simulink library "carnot"  (R2013b)
settings: Solver=ode45  StartTime=0.0  StopTime=10.0  RelTol=1e-3
undefined symbols (not defined in the file or in its folder): A, acol, Ahabit, Awin, Azimuth_Angle, AziWin, B, C, c1, c4, capc, caph, CarnotCallbacks_Density, CarnotCallbacks_Enthalpy, CarnotCallbacks_Enthalpy2Temperature, CarnotCallbacks_Entropy, CarnotCallbacks_Evaporation_Enthalpy, CarnotCallbacks_GlobalMessageLevel, CarnotCallbacks_Grashof, CarnotCallbacks_Heat_Capacity, CarnotCallbacks_Kinematic_Viscosity, CarnotCallbacks_Prandtl, CarnotCallbacks_Saturation_Property, CarnotCallbacks_Saturation_Temperature, CarnotCallbacks_Saturation_Value_Water, CarnotCallbacks_Specific_Volume, CarnotCallbacks_Thermal_Conductivity, CarnotCallbacks_Vapour_Content, CarnotCallbacks_Vapour_Pressure, con, cond, d, Dd, density, dfin, dia, DiameterLastPiece, DPConstant, dpipe, DPLinear, DPQuadratic, emission_out, fluid, FluidMix, FluidType, FPC, frame, g, GeodeticHeight, Gwin, heat_capacity, hgt, HP, Hroom, ID, inlet, K, l, lin, lpipe ... (+29)
undefined symbols (not defined in the file): c2, c3, c5, c6, cwall, dactive, height, mc, mID, rho, tau, UAneighbour, UAwall, uloss
libraries: carnot x333, simulink x25, simulink_extras x7
(part 13 of 16)

== system carnot/Storage/Thermal/Storage_Type_4_CONF ==
  Tamb : Inport
  THB_dhw : Inport  Port=2
  THB_bkpDHW : Inport  Port=3
  THB_hec : Inport  Port=4
  THB_sol : Inport  Port=5
  Storage_Type_4 : carnot/Storage/Thermal/Storage_Type_4  uloss=0.74  ubot=1.37  utop=0.74  cond=0.62  t0=tini  volume=0.75  dia=0.79  pos=standing cylinder  nconnect=4  nodes=50  mpoints=50
  T_Sensor_Surface : carnot/Control/T_Sensor_Surface  pos="[0.2         0.5         0.6]"  tdel=10  t0=tini(1)
  Sdat : Outport
  Tstg : Outport  Port=2
  THBdhw : Outport  Port=3
  THBbkpDHW : Outport  Port=4
  THBhec : Outport  Port=5
  THBsol : Outport  Port=6
  wires:
  Storage_Type_4/2 -> T_Sensor_Surface/1
  Storage_Type_4/1 -> Sdat/1
  THB_sol/1 -> Storage_Type_4/5  "THBsolar_in"
  THB_bkpDHW/1 -> Storage_Type_4/3  "THBbackup_in"
  THB_dhw/1 -> Storage_Type_4/2  "THBdhw_in"
  Tamb/1 -> Storage_Type_4/1
  Storage_Type_4/3 -> THBdhw/1
  Storage_Type_4/4 -> THBbkpDHW/1
  Storage_Type_4/6 -> THBsol/1
  Storage_Type_4/5 -> THBhec/1
  THB_hec/1 -> Storage_Type_4/4
  T_Sensor_Surface/1 -> Tstg/1

== system carnot/Storage/Thermal/Storage_Type_5 ==
  Tamb : Inport
  THB_dhw : Inport  Port=2
  THB_bkDHW : Inport  Port=3
  THB_heating : Inport  Port=4
  THB_bkHT : Inport  Port=5
  THB_solar : Inport  Port=6
  Bus Creator : BusCreator  Inputs=13
  Bus Creator1 : BusCreator  Inputs=2
  Demux : Demux  Outputs=2
  HX_EN12977_dhw : carnot/Storage/Thermal/Storage_Ports/HX_EN12977  h_in=0.02  h_out=0.95  ua0=642.2  uam=0.369  uat=0.684  dplin=100  dpqua=100  nodes=nodes  hgt=height  dia=dia
  HX_EN12977_solar : carnot/Storage/Thermal/Storage_Ports/HX_EN12977  h_in=0.45  h_out=0  ua0=678.6  uam=0.411  uat=0.287  dplin=100  dpqua=100  nodes=nodes  hgt=height  dia=dia
  pipe_bkp_dhw : carnot/Storage/Thermal/Storage_Ports/Pipe  h_in=1  h_out=0.45  nodes=nodes  hgt=height  dia=dia  dplin=10  dpqua=10
  pipe_bkp_heating : carnot/Storage/Thermal/Storage_Ports/Pipe  h_in=0.54  h_out=0.45  nodes=nodes  hgt=height  dia=dia  dplin=10  dpqua=10
  pipe_heating : carnot/Storage/Thermal/Storage_Ports/Pipe  h_in=0.45  h_out=0.54  nodes=nodes  hgt=height  dia=dia  dplin=10  dpqua=10
  select_T : Selector  InputPortWidth=nodes  IndexOptions=Index vector (dialog)  Indices=mpts  OutputSizes=1
  sfun_storageTnodes : carnot/Basic/Thermal_Models/sfun_storageTnodes  dia=dia  volume=volume  standing=standing  uloss=uloss  ubot=utop  utop=ubot  cond=cond  tini=tini  nodes=nodes  nconnect=nconnect
  Sdat : Outport
  T_nodes : Outport  Port=2
  THBdhw : Outport  Port=3
  THBbkDHW : Outport  Port=4
  THBheating : Outport  Port=5
  THBbkHT : Outport  Port=6
  THBsolar : Outport  Port=7
  wires:
  HX_EN12977_solar/2 -> Bus Creator/12, THBsolar/1  "THBsolar_out"
  THB_solar/1 -> Bus Creator/11, HX_EN12977_solar/2  "THBsolar_in"
  Bus Creator1/1 -> Bus Creator/2  "energy"
  Demux/2 -> Bus Creator1/2  "losses"
  Demux/1 -> Bus Creator1/1  "internal"
  pipe_bkp_dhw/1 -> sfun_storageTnodes/3
  pipe_bkp_dhw/2 -> THBbkDHW/1, Bus Creator/10  "THBother_out"
  THB_bkDHW/1 -> pipe_bkp_dhw/2, Bus Creator/9  "THBother_in"
  Bus Creator/1 -> Sdat/1
  sfun_storageTnodes/2 -> select_T/1, pipe_bkp_dhw/1, pipe_heating/1, HX_EN12977_solar/1, pipe_bkp_heating/1, HX_EN12977_dhw/1  "Tnodes"
  sfun_storageTnodes/1 -> Demux/1  "Energy"
  select_T/1 -> Bus Creator/13, T_nodes/1  "Tnodes"
  HX_EN12977_dhw/1 -> sfun_storageTnodes/2
  HX_EN12977_dhw/2 -> Bus Creator/4, THBdhw/1  "THBdhw_out"
  THB_dhw/1 -> Bus Creator/3, HX_EN12977_dhw/2  "THBdhw_in"
  Tamb/1 -> Bus Creator/1, sfun_storageTnodes/1  "Tamb"
  THB_heating/1 -> pipe_heating/2, Bus Creator/5  "THBheating_in"
  pipe_heating/1 -> sfun_storageTnodes/4
  pipe_heating/2 -> THBheating/1, Bus Creator/6  "THBheating_out"
  HX_EN12977_solar/1 -> sfun_storageTnodes/6
  THB_bkHT/1 -> pipe_bkp_heating/2, Bus Creator/7  "THBbackup_in"
  pipe_bkp_heating/1 -> sfun_storageTnodes/5
  pipe_bkp_heating/2 -> THBbkHT/1, Bus Creator/8  "THBbackup_out"

== system carnot/Storage/Thermal/Storage_Type_5_CONF ==
  Tamb : Inport
  THB_dhw : Inport  Port=2
  THB_bkpDHW : Inport  Port=3
  THB_hec : Inport  Port=4
  THB_bkpHec : Inport  Port=5
  THB_sol : Inport  Port=6
  Storage_Type_5 : carnot/Storage/Thermal/Storage_Type_5  uloss=0.74  ubot=1.37  utop=0.74  cond=0.62  t0=tini  volume=0.75  dia=0.79  pos=standing cylinder  nconnect=5  nodes=50  mpoints=50
  T_Sensor_Surface : carnot/Control/T_Sensor_Surface  pos=[0.1 0.5 0.7]  tdel=10  t0=tini(1)
  Sdat : Outport
  Tstg : Outport  Port=2
  THBdhw : Outport  Port=3
  THBbkpDHW : Outport  Port=4
  THBhec : Outport  Port=5
  THBbkpHec : Outport  Port=6
  THBsol : Outport  Port=7
  wires:
  T_Sensor_Surface/1 -> Tstg/1
  THB_bkpHec/1 -> Storage_Type_5/5
  Storage_Type_5/7 -> THBsol/1
  Storage_Type_5/4 -> THBbkpDHW/1
  Storage_Type_5/3 -> THBdhw/1
  Tamb/1 -> Storage_Type_5/1
  THB_dhw/1 -> Storage_Type_5/2  "THBdhw_in"
  THB_bkpDHW/1 -> Storage_Type_5/3  "THBbackup_in"
  THB_sol/1 -> Storage_Type_5/6  "THBsolar_in"
  Storage_Type_5/1 -> Sdat/1
  Storage_Type_5/2 -> T_Sensor_Surface/1
  Storage_Type_5/5 -> THBhec/1
  Storage_Type_5/6 -> THBbkpHec/1
  THB_hec/1 -> Storage_Type_5/4

== system carnot/Storage/Thermal/detailed_storage_models ==
  heat_exchanger_storage : Subsystem  mask(storage with heat exchanger){v=[0.002 0.0005], loss=0.1, uh=[500 1], uc=[500 1], uw=[300 1], mat=aluminium, m=[3 0.1], t0=20, dph=[200 100 1], dpc=[20 10 0.5], n=1}
      mask prompts: v "volume [exchanger storage] [m³]"; loss "ua losses [W/K]"; uh "heat transfer in exchanger [constant linear_in_massflow] [W/K]"; uc "heat transfer to storage [constant linear_massflow] [W/K]"; uw "heat transfer to wall [constant linear_in_massflow] [W/K]"; mat "material"; m "[mass_in_kg fraction_exchanger]"; t0 "initial temperature [degree centigrade]"; dph "pressure drop exchanger [linear quadratic lin_T] [Pa]"; dpc "pressure drop storage [linear quadratic lin_T] [Pa]"; n "number of nodes"
      mask help: This block is a heat exchanger, taking the fluid volume of the cold and hot side and the thermal capacity of the walls into account.
      mask init:
      | v = max(0.00001, v);
      | n = max(n,1);
      mask Help: web(fullfile(path_carnot('help'),'heat_exchanger_storage.html'),'-helpbrowser')
      mask TypeOptions mat: aluminium | bronze | cast iron | steel | stainless steel | copper | brass | gravel | granite | glass | PU-foam | glass wool
      mask Display: plot(0,-10,110,95,[30,30,35,65,70,70,65,35,30],[90,60,54,54,60,90,95,95,90],[30,66,34,66,34,66,30],[63,63,68,73,76,81,81])

== system carnot/Storage/Thermal/surface_models ==
  Isolated_Cover : Subsystem  mask(isolated cover){u=0.6}
      mask prompts: u "loss coefficient of isolation [W/(m²*K)]"
      mask help: This is a surface-model for ground storages. It describes the absorption of solar radiation and the heat losses by wind.
      mask Help: web(fullfile(path_carnot('help'),'Isolated_Cover.html'),'-helpbrowser')
  Open_Surface : Subsystem  mask(open surface){albedo=0.6}
      mask prompts: albedo "albedo of the surface [0..1]"
      mask help: This is a surface-model for ground storages. It describes the absorption of solar radiation and the heat losses by wind.
      mask init:
      | albedo = min(1, max(0, albedo));
      mask Help: web(fullfile(path_carnot('help'),'Open_Surface.html'),'-helpbrowser')

== system carnot/Basic/Hydraulics/Flow_Mixer_basic/average_1 ==
  In1 : Inport
  In2 : Inport  Port=2
  average2 : Gain  Gain=0.5  SaturateOnIntegerOverflow=on  OutDataTypeStr=Inherit: Same as input  ParamDataTypeStr=Inherit: Same as input
  sum2 : Sum  SaturateOnIntegerOverflow=on  InputSameDT=on  OutDataTypeStr=Inherit: Same as first input
  Out1 : Outport
  wires:
  In1/1 -> sum2/1
  average2/1 -> Out1/1
  sum2/1 -> average2/1
  In2/1 -> sum2/2

== system carnot/Basic/Hydraulics/Flow_Mixer_basic/decrease_ID1 ==
  In1 : Inport
  Abs : Abs
  Bias : Bias  Bias=-1
  Dot Product1 : DotProduct  InputSameDT=on  OutDataTypeStr=Inherit: Inherit via internal rule
  Sign : Signum
  Out1 : Outport
  wires:
  Bias/1 -> Dot Product1/2
  Sign/1 -> Dot Product1/1
  Abs/1 -> Bias/1
  Dot Product1/1 -> Out1/1
  In1/1 -> Sign/1, Abs/1

== system carnot/Basic/Hydraulics/Flow_Mixer_basic/decrease_ID2 ==
  In1 : Inport
  Abs : Abs
  Bias : Bias  Bias=-1
  Dot Product1 : DotProduct  InputSameDT=on  OutDataTypeStr=Inherit: Inherit via internal rule
  Sign : Signum
  Out1 : Outport
  wires:
  In1/1 -> Abs/1, Sign/1
  Dot Product1/1 -> Out1/1
  Abs/1 -> Bias/1
  Sign/1 -> Dot Product1/1
  Bias/1 -> Dot Product1/2

== system carnot/Basic/Hydraulics/Mix_T_Mdot/select1 ==
  In1 : Inport
  Bus Selector1 : BusSelector  OutputSignals=Temperature,MassFlow,Pressure,FluidType,FluidMix
  Mux : Mux  Inputs=5
  Out1 : Outport
  wires:
  Mux/1 -> Out1/1
  In1/1 -> Bus Selector1/1
  Bus Selector1/5 -> Mux/5  "<FluidMix>"
  Bus Selector1/4 -> Mux/4  "<FluidType>"
  Bus Selector1/3 -> Mux/3  "<Pressure>"
  Bus Selector1/2 -> Mux/2  "<MassFlow>"
  Bus Selector1/1 -> Mux/1  "<Temperature>"

== system carnot/Basic/Hydraulics/Mix_T_Mdot/select2 ==
  In1 : Inport
  Bus Selector1 : BusSelector  OutputSignals=Temperature,MassFlow,Pressure,FluidType,FluidMix
  Mux : Mux  Inputs=5
  Out1 : Outport
  wires:
  Bus Selector1/1 -> Mux/1  "<Temperature>"
  Bus Selector1/2 -> Mux/2  "<MassFlow>"
  Bus Selector1/3 -> Mux/3  "<Pressure>"
  Bus Selector1/4 -> Mux/4  "<FluidType>"
  Bus Selector1/5 -> Mux/5  "<FluidMix>"
  In1/1 -> Bus Selector1/1
  Mux/1 -> Out1/1

== system carnot/Basic/Pressure_Drop/Pressure_Drop_Fix/c_calc ==
  Enable : EnablePort
  Constant : Constant  Value=con
  con : Outport  InitialOutput=con
  wires:
  Constant/1 -> con/1

== system carnot/Basic/Pressure_Drop/Pressure_Drop_Fix/lq_calc ==
  Enable : EnablePort
  Constant : Constant  Value=lin
  Constant1 : Constant  Value=qua
  Out1 : Outport  InitialOutput=lin
  Out2 : Outport  Port=2  InitialOutput=qua
  wires:
  Constant/1 -> Out1/1
  Constant1/1 -> Out2/1

== system carnot/Basic/Pressure_Drop/Pressure_Drop_PipeTheory/DP_Geometry ==
  Tnodes : Inport
  mdot : Inport  Port=2
  Enable : EnablePort
  Bus Selector4 : BusSelector  OutputSignals=MassFlow,Pressure,FluidType,FluidMix
  S-Function : S-Function  FunctionName=pipe_PressureDrop  Parameters="dia, len,  rough, nbend"  EnableBusSupport=off
  lin : Outport  OutputWhenDisabled=reset  InitialOutput=0
  qua : Outport  Port=2  OutputWhenDisabled=reset  InitialOutput=0
  dp : Outport  Port=3  OutputWhenDisabled=reset  InitialOutput=0
  wires:
  Tnodes/1 -> S-Function/1
  S-Function/1 -> lin/1
  S-Function/2 -> qua/1
  mdot/1 -> Bus Selector4/1
  Bus Selector4/1 -> S-Function/2  "<MassFlow>"
  Bus Selector4/2 -> S-Function/3  "<Pressure>"
  Bus Selector4/3 -> S-Function/4  "<FluidType>"
  Bus Selector4/4 -> S-Function/5  "<FluidMix>"
  S-Function/3 -> dp/1

== system carnot/Basic/Pressure_Drop/Pressure_Drop_changeD/2//pi//d^2//density ==
  note: dp = ceta * density/2 *v^2
      | for Dlast > Dhere : ceta = (1 - D_last/D_here)^2
      | v = mdot/A/density
      | dp = ceta * mdot^2 / 2 / A^2 / densitiy
      | with A = pi/4*d^2
      | dp = 8*mdot^2/pi^2/d^4/denstiy
      | dp=qua*mdot^2
      | qua = 8/(pi^2*density) * ceta / d^4
  THB : Inport
  Enable : EnablePort
  Bus Selector3 : BusSelector  OutputSignals=DiameterLastPiece
  Density : carnot/Basic/Material_Properties/Density  VariantControl=CarlibClassic  INPUTARGUMENTS=THB  DEBUGLEVEL=DEBUGLEVEL  MAXTOTALWARNINGS=inf  MAXCONSECUTIVEWARNINGS=inf  WRITETOFILE=0  FILENAME='errors.txt'
  Gain : Gain  Gain=pi^2/8
  Gain1 : Gain  Gain=1/dia
  Lookup Table : Lookup  InputValues=[0:0.05:1, 10, 100]  Table="[(1 - [0:0.05:1]).^2,  1.2, 1.2]"
  Math Function2 : Math  Operator=square  SaturateOnIntegerOverflow=on
  Math Function3 : Math  Operator=square  SaturateOnIntegerOverflow=on
  Product : Product  Inputs=/*/  RndMeth=Zero
  min(Dlast,dia) : Saturate  UpperLimit=dia  LowerLimit=0
  qua : Outport
  wires:
  Density/1 -> Gain/1
  THB/1 -> Bus Selector3/1, Density/1
  Bus Selector3/1 -> Gain1/1, min(Dlast,dia)/1  "<DiameterLastPiece>"
  Gain/1 -> Product/1
  Product/1 -> qua/1
  Gain1/1 -> Lookup Table/1  "Dlast/D"
  min(Dlast,dia)/1 -> Math Function2/1
  Math Function2/1 -> Math Function3/1
  Math Function3/1 -> Product/3
  Lookup Table/1 -> Product/2  "ceta"

== system carnot/Basic/Pressure_Drop/Pressure_Drop_staticHeight/Density_x_Gravity ==
  Tnodes : Inport
  THB : Inport  Port=2
  height : Inport  Port=3
  Enable : EnablePort
  Add : Sum
  Add1 : Sum  Inputs=1
  Bus Selector4 : BusSelector  OutputSignals=Pressure,FluidType,FluidMix,GeodeticHeight
  Constant : Constant  Value=9.81
  Density : carnot/Basic/Material_Properties/Density  VariantControl=CarlibClassic  INPUTARGUMENTS=state variables (classic)  DEBUGLEVEL=DEBUGLEVEL  MAXTOTALWARNINGS=inf  MAXCONSECUTIVEWARNINGS=inf  WRITETOFILE=0  FILENAME='errors.txt'
  Product : Product  Inputs=/***  RndMeth=Zero
  Width : Width
  pstat : Outport
  GeodeticHeight : Outport  Port=2
  wires:
  Add1/1 -> pstat/1
  Constant/1 -> Product/3
  Product/1 -> Add1/1
  Density/1 -> Product/4
  Width/1 -> Product/1
  Add/1 -> GeodeticHeight/1
  height/1 -> Product/2, Add/2
  Bus Selector4/4 -> Add/1  "<GeodeticHeight>"
  Tnodes/1 -> Width/1, Density/1
  THB/1 -> Bus Selector4/1
  Bus Selector4/3 -> Density/4  "<FluidMix>"
  Bus Selector4/2 -> Density/3  "<FluidType>"
  Bus Selector4/1 -> Density/2  "<Pressure>"

== system carnot/Basic/Thermal_Models/Combustion_Calculation/exhaust gas ==
  note: gas = 1
      | liquid = 2
      | solid = 3
  ID : Inport
  h : Inport  Port=2
  c : Inport  Port=3
  o : Inport  Port=4
  s : Inport  Port=5
  n : Inport  Port=6
  w : Inport  Port=7
  Demux : Demux
  Multiport Switch : MultiPortSwitch  SaturateOnIntegerOverflow=on  InputSameDT=on
  Terminator : Terminator
  fluid/solid : Subsystem
  gas : Subsystem
  CO2 : Outport
  H2O : Outport  Port=2
  SO2 : Outport  Port=3
  N2 : Outport  Port=4
  wires:
  ID/1 -> Multiport Switch/1
  fluid/solid/1(Out1) -> Multiport Switch/4, Multiport Switch/3
  Multiport Switch/1 -> Demux/1
  Demux/4 -> N2/1
  Demux/3 -> SO2/1
  Demux/2 -> H2O/1
  Demux/1 -> CO2/1
  s/1 -> gas/3(s), fluid/solid/3(s)
  n/1 -> gas/4(n), fluid/solid/4(n)
  h/1 -> gas/2(h), fluid/solid/2(h)
  c/1 -> gas/1(c), fluid/solid/1(c)
  o/1 -> Terminator/1
  w/1 -> fluid/solid/5(w)
  gas/1(Out1) -> Multiport Switch/2

== system carnot/Basic/Thermal_Models/HeatPump_basic/P_el calculus ==
  note: Pel = K4*Tcold_in + K5*Thot_out + K6
  Thot_out : Inport
  Tcold_in : Inport  Port=2
  Add : Sum  Inputs=+++
  Thot_dependancy : Gain  Gain=K(5)  SaturateOnIntegerOverflow=on  OutDataTypeStr=Inherit: Same as input  ParamDataTypeStr=Inherit: Same as input
  Tsource dependancy : Gain  Gain=K(4)  SaturateOnIntegerOverflow=on  OutDataTypeStr=Inherit: Same as input  ParamDataTypeStr=Inherit: Same as input
  constant power : Constant  Value=K(6)
  P_el : Outport
  wires:
  Thot_dependancy/1 -> Add/1
  Thot_out/1 -> Thot_dependancy/1
  Tsource dependancy/1 -> Add/2
  Add/1 -> P_el/1
  Tcold_in/1 -> Tsource dependancy/1
  constant power/1 -> Add/3

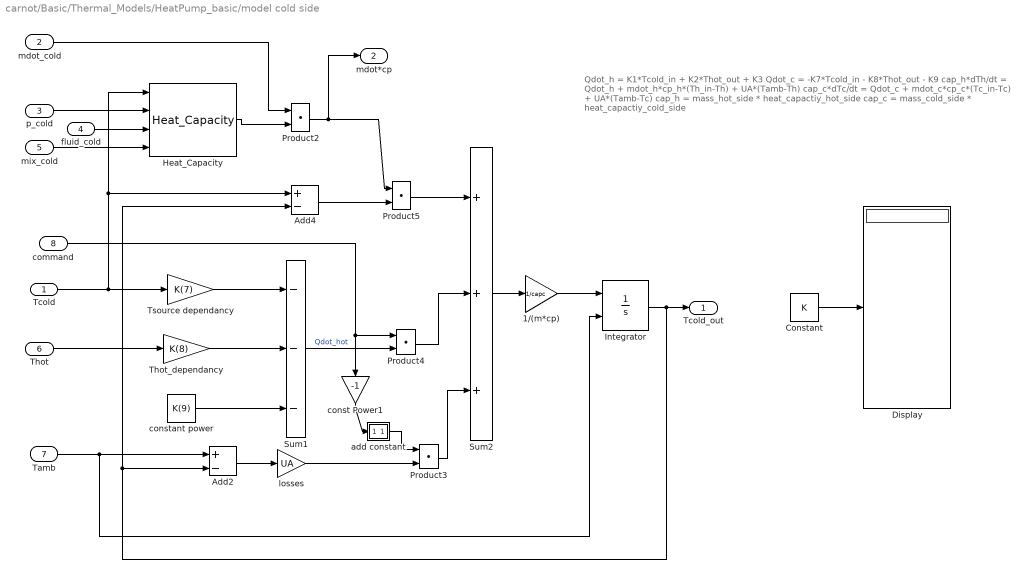
== system carnot/Basic/Thermal_Models/HeatPump_basic/model cold side ==
  note: Qdot_h = K1*Tcold_in + K2*Thot_out + K3
      |
      | Qdot_c = -K7*Tcold_in - K8*Thot_out - K9
      |
      | cap_h*dTh/dt = Qdot_h + mdot_h*cp_h*(Th_in-Th) + UA*(Tamb-Th)
      |
      | cap_c*dTc/dt = Qdot_c + mdot_c*cp_c*(Tc_in-Tc) + UA*(Tamb-Tc)
      |
      | cap_h = mass_hot_side * heat_capactiy_hot_side
      |
      | cap_c = mass_cold_side * heat_capactiy_cold_side
  Tcold : Inport
  mdot_cold : Inport  Port=2
  p_cold : Inport  Port=3
  fluid_cold : Inport  Port=4
  mix_cold : Inport  Port=5
  Thot : Inport  Port=6
  Tamb : Inport  Port=7
  command : Inport  Port=8
  1/(m*cp) : Gain  Gain=1/capc
  Add2 : Sum  Inputs=+-
  Add4 : Sum  Inputs=+-
  Constant : Constant  Value=K
  Display : Display
  Heat_Capacity : carnot/Basic/Material_Properties/Heat_Capacity  VariantControl=CarlibClassic  INPUTARGUMENTS=state variables (classic)  DEBUGLEVEL=DEBUGLEVEL  MAXTOTALWARNINGS=inf  MAXCONSECUTIVEWARNINGS=inf  WRITETOFILE=0  FILENAME='errors.txt'
  Integrator : Integrator  InitialConditionSource=external  InitialCondition=25
  Product{2..5} (4 alike) : DotProduct  InputSameDT=on  OutDataTypeStr=Inherit: Inherit via internal rule
  Sum1 : Sum  Inputs=---  SaturateOnIntegerOverflow=on  InputSameDT=on  OutDataTypeStr=Inherit: Same as first input
  Sum2 : Sum  Inputs=3  SaturateOnIntegerOverflow=on  InputSameDT=on  OutDataTypeStr=Inherit: Same as first input
  Thot_dependancy : Gain  Gain=K(8)  SaturateOnIntegerOverflow=on  OutDataTypeStr=Inherit: Same as input  ParamDataTypeStr=Inherit: Same as input
  Tsource dependancy : Gain  Gain=K(7)  SaturateOnIntegerOverflow=on  OutDataTypeStr=Inherit: Same as input  ParamDataTypeStr=Inherit: Same as input
  add constant : Subsystem  mask(add constant){c=+1}
      mask prompts: c "constant c"
      mask help: This block adds a constant c to each element of the input vector.
      mask Help: eval('htmlhelp (''chap_4_2a.htm#add_constant'')')
      mask Display: disp('+c');
  const Power1 : Gain  Gain=-1  SaturateOnIntegerOverflow=on  OutDataTypeStr=Inherit: Same as input  ParamDataTypeStr=Inherit: Same as input
  constant power : Constant  Value=K(9)
  losses : Gain  Gain=UA
  Tcold_out : Outport
  mdot*cp : Outport  Port=2
  wires:
  Constant/1 -> Display/1
  1/(m*cp)/1 -> Integrator/1
  fluid_cold/1 -> Heat_Capacity/3
  mix_cold/1 -> Heat_Capacity/4
  p_cold/1 -> Heat_Capacity/2
  Thot/1 -> Thot_dependancy/1
  Product2/1 -> mdot*cp/1, Product5/1
  Heat_Capacity/1 -> Product2/2
  mdot_cold/1 -> Product2/1
  Add2/1 -> losses/1
  Tcold/1 -> Add4/1, Heat_Capacity/1, Tsource dependancy/1
  Tsource dependancy/1 -> Sum1/1
  Thot_dependancy/1 -> Sum1/2
  constant power/1 -> Sum1/3
  Sum1/1 -> Product4/2  "Qdot_hot"
  Tamb/1 -> Add2/1, Integrator/2
  command/1 -> Product4/1, const Power1/1
  losses/1 -> Product3/2
  add constant/1(Out1) -> Product3/1
  const Power1/1 -> add constant/1(In1)
  Add4/1 -> Product5/2
  Sum2/1 -> 1/(m*cp)/1
  Product3/1 -> Sum2/3
  Product4/1 -> Sum2/2
  Product5/1 -> Sum2/1
  Integrator/1 -> Tcold_out/1, Add2/2, Add4/2

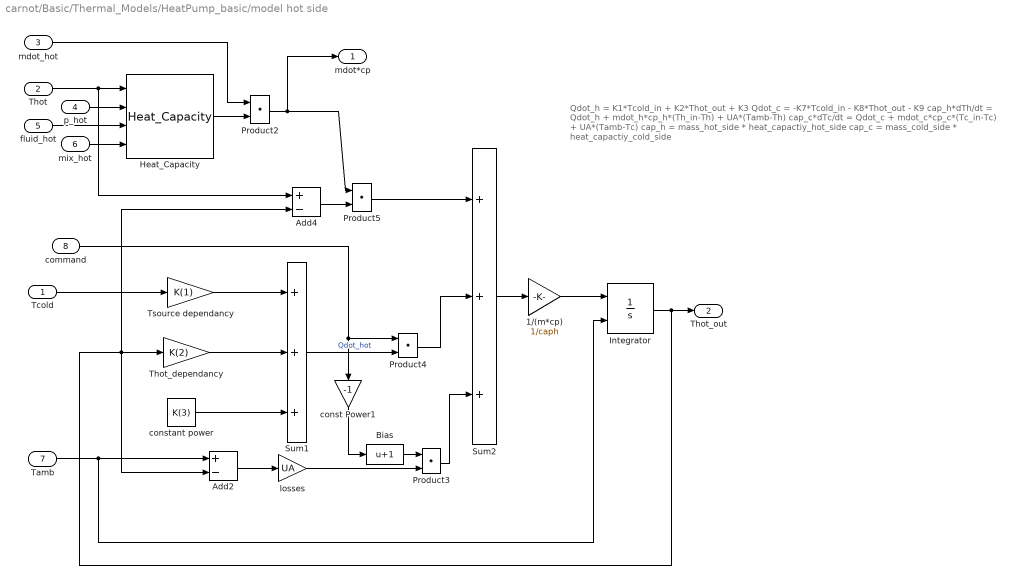
== system carnot/Basic/Thermal_Models/HeatPump_basic/model hot side ==
  note: Qdot_h = K1*Tcold_in + K2*Thot_out + K3
      |
      | Qdot_c = -K7*Tcold_in - K8*Thot_out - K9
      |
      | cap_h*dTh/dt = Qdot_h + mdot_h*cp_h*(Th_in-Th) + UA*(Tamb-Th)
      |
      | cap_c*dTc/dt = Qdot_c + mdot_c*cp_c*(Tc_in-Tc) + UA*(Tamb-Tc)
      |
      | cap_h = mass_hot_side * heat_capactiy_hot_side
      |
      | cap_c = mass_cold_side * heat_capactiy_cold_side
  Tcold : Inport
  Thot : Inport  Port=2
  mdot_hot : Inport  Port=3
  p_hot : Inport  Port=4
  fluid_hot : Inport  Port=5
  mix_hot : Inport  Port=6
  Tamb : Inport  Port=7
  command : Inport  Port=8
  1/(m*cp) : Gain  Gain=1/caph
  Add2 : Sum  Inputs=+-
  Add4 : Sum  Inputs=+-
  Bias : Bias  Bias=1
  Heat_Capacity : carnot/Basic/Material_Properties/Heat_Capacity  VariantControl=CarlibClassic  INPUTARGUMENTS=state variables (classic)  DEBUGLEVEL=DEBUGLEVEL  MAXTOTALWARNINGS=inf  MAXCONSECUTIVEWARNINGS=inf  WRITETOFILE=0  FILENAME='errors.txt'
  Integrator : Integrator  InitialConditionSource=external  InitialCondition=25
  Product{2..5} (4 alike) : DotProduct  InputSameDT=on  OutDataTypeStr=Inherit: Inherit via internal rule
  Sum1 : Sum  Inputs=+++  SaturateOnIntegerOverflow=on  InputSameDT=on  OutDataTypeStr=Inherit: Same as first input
  Sum2 : Sum  Inputs=+++  SaturateOnIntegerOverflow=on  InputSameDT=on  OutDataTypeStr=Inherit: Same as first input
  Thot_dependancy : Gain  Gain=K(2)  SaturateOnIntegerOverflow=on  OutDataTypeStr=Inherit: Same as input  ParamDataTypeStr=Inherit: Same as input
  Tsource dependancy : Gain  Gain=K(1)  SaturateOnIntegerOverflow=on  OutDataTypeStr=Inherit: Same as input  ParamDataTypeStr=Inherit: Same as input
  const Power1 : Gain  Gain=-1  SaturateOnIntegerOverflow=on  OutDataTypeStr=Inherit: Same as input  ParamDataTypeStr=Inherit: Same as input
  constant power : Constant  Value=K(3)
  losses : Gain  Gain=UA
  mdot*cp : Outport
  Thot_out : Outport  Port=2
  wires:
  Integrator/1 -> Add2/2, Thot_dependancy/1, Add4/2, Thot_out/1
  Product5/1 -> Sum2/1
  Product4/1 -> Sum2/2
  Product3/1 -> Sum2/3
  1/(m*cp)/1 -> Integrator/1
  Sum2/1 -> 1/(m*cp)/1
  Add4/1 -> Product5/2
  const Power1/1 -> Bias/1
  Bias/1 -> Product3/1
  losses/1 -> Product3/2
  command/1 -> const Power1/1, Product4/1
  Tamb/1 -> Integrator/2, Add2/1
  Sum1/1 -> Product4/2  "Qdot_hot"
  constant power/1 -> Sum1/3
  Thot_dependancy/1 -> Sum1/2
  Tsource dependancy/1 -> Sum1/1
  Tcold/1 -> Tsource dependancy/1
  Add2/1 -> losses/1
  mdot_hot/1 -> Product2/1
  Heat_Capacity/1 -> Product2/2
  Product2/1 -> Product5/1, mdot*cp/1
  Thot/1 -> Add4/1, Heat_Capacity/1
  p_hot/1 -> Heat_Capacity/2
  mix_hot/1 -> Heat_Capacity/4
  fluid_hot/1 -> Heat_Capacity/3

== system carnot/Basic/Thermal_Models/House_OneNodeModel/troom_calc ==
  Qdot : Inport
  1/mc : Gain  Gain=invmc  SaturateOnIntegerOverflow=on  OutDataTypeStr=Inherit: Same as input  ParamDataTypeStr=Inherit: Same as input
  Switch : Switch  Criteria=u2 > Threshold
  const : Constant  Value=tini
  dtroom : Constant  Value=dtroom
  energy : Integrator  InitialCondition=tini  LimitOutput=on  UpperSaturationLimit=tini+max(0.01,dtroom)  LowerSaturationLimit=tini-max(0.01,dtroom)
  sum : Sum  Inputs=1  SaturateOnIntegerOverflow=on  InputSameDT=on  OutDataTypeStr=Inherit: Same as first input
  Troom : Outport
  wires:
  Qdot/1 -> sum/1
  dtroom/1 -> Switch/2
  Switch/1 -> Troom/1  "Troom"
  energy/1 -> Switch/1
  1/mc/1 -> energy/1
  sum/1 -> 1/mc/1
  const/1 -> Switch/3

== system carnot/Basic/Thermal_Models/Radiator_basic/Transfer Fcn (with initial states) ==
  In1 : Inport
  State Space : StateSpace  A=A  B=B  C=C  D=Dd  X0=X0
  Out1 : Outport  InitialOutput=0
  wires:
  State Space/1 -> Out1/1
  In1/1 -> State Space/1

== system carnot/Load/Hot_Water_Tapping/Applications/Hot_Water_Consumption_EN13203 ==
  THBhot : Inport
  DHW_Energy_Tapping : Reference
  T_cold_water_const : Constant  Value=10
  Water_Tap : Reference
  flow_diverter : Reference
  flow_mixer_thermostatic : Reference
  THBcold : Outport  InitialOutput=0
  THBwarm : Outport  Port=2
  Tset : Outport  Port=3  InitialOutput=0
  wires:
  DHW_Energy_Tapping/1 -> Water_Tap/1
  T_cold_water_const/1 -> DHW_Energy_Tapping/1, Water_Tap/2
  Water_Tap/1 -> flow_diverter/1
  flow_mixer_thermostatic/2 -> flow_diverter/2
  flow_mixer_thermostatic/1 -> THBwarm/1
  THBhot/1 -> flow_mixer_thermostatic/1
  flow_diverter/1 -> THBcold/1
  flow_diverter/2 -> flow_mixer_thermostatic/2
  flow_diverter/3 -> flow_mixer_thermostatic/3
  DHW_Energy_Tapping/2 -> Tset/1, flow_mixer_thermostatic/4

== system carnot/Load/Hot_Water_Tapping/Applications/Hot_Water_Consumption_basic ==
  THBhot : Inport
  T_cold_water_const : Constant  Value=10
  T_hot_water : Constant  Value=45
  Water_Tap : Reference
  flow_diverter : Reference
  flow_mixer_thermostatic : Reference
  mdot_40_20_40 : Reference
  THBcold : Outport  InitialOutput=0
  THBwarm : Outport  Port=2
  Tset : Outport  Port=3  InitialOutput=0
  wires:
  flow_diverter/3 -> flow_mixer_thermostatic/3
  flow_diverter/2 -> flow_mixer_thermostatic/2
  flow_diverter/1 -> THBcold/1
  THBhot/1 -> flow_mixer_thermostatic/1
  flow_mixer_thermostatic/1 -> THBwarm/1
  flow_mixer_thermostatic/2 -> flow_diverter/2
  Water_Tap/1 -> flow_diverter/1
  T_hot_water/1 -> Tset/1, flow_mixer_thermostatic/4
  T_cold_water_const/1 -> Water_Tap/2
  mdot_40_20_40/1 -> Water_Tap/1

== system carnot/Load/Houses/Simple_House_ISO_GroundModel/Internal_Gain_Profile ==
  Electric_Gains_Profile : carnot/Load/General/Repeating_Profile  period=24*3600  rep_seq_t=[0 1 6 7 8 9 11 12 13 18 19 20 22 23]*3600  rep_seq_d=[1 5 1 1 1 2 1 1 4 2 1 2 1 1]*3600  rep_seq_y=[105 55 392.5 457.5 420 55 250 55 120 170 615 420 442.5 355]
  Mux1 : Mux  Inputs=2
  Occupation_Profile : carnot/Load/General/Repeating_Profile  period=24*3600  rep_seq_t=[0 6 7 8 9 11 12 13 14 15 17 18 20 21 22]*3600  rep_seq_d=[6 1 1 1 2 1 1 1 1 2 1 2 1 1 2]*3600  rep_seq_y=[4 2 3 2 0 1 3 2 1 0 1 2 4 3 4]*60
  Sum: Internal load profile : Sum  Inputs=+
  Internal_Gain : Outport
  wires:
  Mux1/1 -> Sum: Internal load profile/1
  Occupation_Profile/1 -> Mux1/1
  Electric_Gains_Profile/1 -> Mux1/2
  Sum: Internal load profile/1 -> Internal_Gain/1

== system carnot/Load/Houses/Simple_House_ISO_GroundModel/Shading_Control ==
  WDB : Inport
  Troom : Inport  Port=2
  10 minutes lowpass : TransferFcn  Denominator=[600 1]
  Bus Selector : BusSelector  OutputSignals=Temperature_Ambient
  Bus Selector1 : BusSelector  OutputSignals=Solar_Radiation_direct_surface,Solar_Radiation_diffuse_surface  OutputAsBus=on
  Compare To Constant : simulink/Logic and Bit Operations/Compare To Constant  relop=>=  const=10  OutDataTypeStr=uint8
  Direct Lookup Table (n-D) : LookupNDDirect  NumberOfTableDimensions=1  Table=[1 1-shade]
  Logical Operator : Logic  Inputs=3  AllPortsSameDT=off  OutDataTypeStr=boolean
  Relay : Relay  OnSwitchValue=300  OffSwitchValue=200  OutDataTypeStr=uint8
  Relay1 : Relay  OnSwitchValue=23.8  OffSwitchValue=22.8  OutDataTypeStr=uint8
  Sum of Elements : Sum  Inputs=+
  Shading : Outport
  wires:
  Bus Selector1/1 -> Sum of Elements/1
  10 minutes lowpass/1 -> Compare To Constant/1
  Logical Operator/1 -> Direct Lookup Table (n-D)/1
  Sum of Elements/1 -> Relay/1
  Relay/1 -> Logical Operator/2
  Compare To Constant/1 -> Logical Operator/3
  Troom/1 -> Relay1/1
  Direct Lookup Table (n-D)/1 -> Shading/1
  WDB/1 -> Bus Selector1/1, Bus Selector/1
  Relay1/1 -> Logical Operator/1
  Bus Selector/1 -> 10 minutes lowpass/1  "<Temperature_Ambient>"

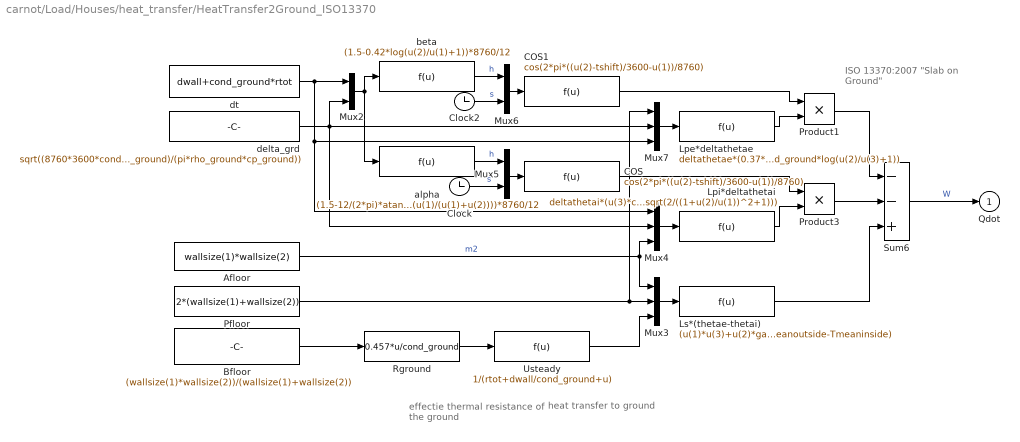
== system carnot/Load/Houses/heat_transfer/HeatTransfer2Ground_ISO13370 ==
  note: heat transfer
      | to ground
  note: effectie thermal resistance
      | of the ground
  note: ISO 13370:2007 "Slab on Ground"
  Afloor : Constant  Value=wallsize(1)*wallsize(2)
  Bfloor : Constant  Value=(wallsize(1)*wallsize(2))/(wallsize(1)+wallsize(2))
  COS : Fcn  Expr=cos(2*pi*((u(2)-tshift)/3600-u(1))/8760)
  COS1 : Fcn  Expr=cos(2*pi*((u(2)-tshift)/3600-u(1))/8760)
  Clock : Clock
  Clock2 : Clock
  Lpe*deltathetae : Fcn  Expr=deltathetae*(0.37*u(1)*cond_ground*log(u(2)/u(3)+1))
  Lpi*deltathetai : Fcn  Expr=deltathetai*(u(3)*cond_ground/u(1)*sqrt(2/((1+u(2)/u(1))^2+1)))
  Ls*(thetae-thetai) : Fcn  Expr=(u(1)*u(3)+u(2)*gammat)*(Tmeanoutside-Tmeaninside)
  Mux2 : Mux  Inputs=2
  Mux3 : Mux  Inputs=3
  Mux4 : Mux  Inputs=3
  Mux5 : Mux  Inputs=2
  Mux6 : Mux  Inputs=2
  Mux7 : Mux  Inputs=3
  Pfloor : Constant  Value=2*(wallsize(1)+wallsize(2))
  Product1 : Product  SaturateOnIntegerOverflow=on  RndMeth=Zero  InputSameDT=on  OutDataTypeStr=Inherit: Same as first input
  Product3 : Product  SaturateOnIntegerOverflow=on  RndMeth=Zero  InputSameDT=on  OutDataTypeStr=Inherit: Same as first input
  Rground : Fcn  Expr=0.457*u/cond_ground
  Sum6 : Sum  Inputs=--+
  Usteady : Fcn  Expr=1/(rtot+dwall/cond_ground+u)
  alpha : Fcn  Expr=(1.5-12/(2*pi)*atan(u(1)/(u(1)+u(2))))*8760/12
  beta : Fcn  Expr=(1.5-0.42*log(u(2)/u(1)+1))*8760/12
  delta_grd : Constant  Value=sqrt((8760*3600*cond_ground)/(pi*rho_ground*cp_ground))
  dt : Constant  Value=dwall+cond_ground*rtot
  Qdot : Outport  InitialOutput=0
  wires:
  Rground/1 -> Usteady/1
  Bfloor/1 -> Rground/1
  dt/1 -> Mux2/1, Mux4/1, Mux7/3
  delta_grd/1 -> Mux4/2, Mux7/2, Mux2/2
  Mux2/1 -> alpha/1, beta/1
  Mux3/1 -> Ls*(thetae-thetai)/1
  Afloor/1 -> Mux4/3, Mux3/1  "m2"
  Pfloor/1 -> Mux3/2, Mux7/1
  Usteady/1 -> Mux3/3
  Mux4/1 -> Lpi*deltathetai/1
  Lpi*deltathetai/1 -> Product3/2
  alpha/1 -> Mux5/1  "h"
  Clock/1 -> Mux5/2  "s"
  Mux5/1 -> COS/1
  COS/1 -> Product3/1
  Product3/1 -> Sum6/2
  Ls*(thetae-thetai)/1 -> Sum6/3
  beta/1 -> Mux6/1  "h"
  Clock2/1 -> Mux6/2  "s"
  Mux6/1 -> COS1/1
  COS1/1 -> Product1/1
  Lpe*deltathetae/1 -> Product1/2
  Product1/1 -> Sum6/1
  Mux7/1 -> Lpe*deltathetae/1
  Sum6/1 -> Qdot/1  "W"

== system carnot/Load/Houses/heat_transfer/HeatTransfer2Ground_Simple ==
  Troom : Inport
  Sum2 : Sum  Inputs=+-  SaturateOnIntegerOverflow=on  InputSameDT=on  OutDataTypeStr=Inherit: Same as first input
  UAground : Gain  Gain=UAground  SaturateOnIntegerOverflow=on  OutDataTypeStr=Inherit: Same as input  ParamDataTypeStr=Inherit: Same as input
  const1 : Constant  Value=Tground
  Qdot : Outport
  wires:
  Sum2/1 -> UAground/1
  const1/1 -> Sum2/1
  UAground/1 -> Qdot/1
  Troom/1 -> Sum2/2

== system carnot/Load/Houses/heat_transfer/alfa_ceiling ==
  note: (°C)
  note: (W/m^2)
  note: Convective and radiative heat transfer at the SURFACE OF A HORIZONTAL CEILING
  note: s: surface
      | c: convective
      | r: radiative
  note: CONVENTION:
      | Qdot > 0 and qdots < 0, if Ts > T (heat flows from wall surface to room node),
      | Qdot < 0 and qdots > 0, if Ts < T (heat flows from room node to wall surface).
  note: dynamic, convective heat transfer coefficients according to: Glück B.: Wärmeübergangskoeffizienten an thermisch aktiven Bauteiloberflächen
      | und der Übergang zu Basiskennlinien für die Wärmestromdichte; gi Gesundheits-Ingenieur; 128. Jahrgang 2007, Heft 1, Seiten 1-10
  Ts : Inport
  "[AIV]c" : Inport  Port=2
  1-D Lookup Table : Lookup_n-D  NumberOfTableDimensions=1  BreakpointsForDimension1=[-10 -0.01 0.01 10]  BeginIndexSearchUsingPreviousIndexResult=on  Table=[2 2 0.54 0.54]  InternalRulePriority=Speed  RndMeth=Simplest  InputSameDT=on
  Abs : Abs
  Constant : Constant  Value=0.31
  Demux : Demux  Outputs=[1 1 1 6]
  Ground : Ground
  Ground1 : Ground
  Ground2 : Ground
  Math Function : Math  Operator=pow  SaturateOnIntegerOverflow=on
  Mux : Mux  Inputs=[1 1]
  Mux1 : Mux  Inputs=[4 1 1 2 5]
  Product1 : Product  Inputs=3  SaturateOnIntegerOverflow=on  RndMeth=Zero  InputSameDT=on  OutDataTypeStr=Inherit: Same as first input
  Sum : Sum  Inputs=-+  SaturateOnIntegerOverflow=on  InputSameDT=on  OutDataTypeStr=Inherit: Same as first input
  Sum1 : Sum  Inputs=+-  SaturateOnIntegerOverflow=on  InputSameDT=on  OutDataTypeStr=Inherit: Same as first input
  Sum2 : Sum  Inputs=--  SaturateOnIntegerOverflow=on  InputSameDT=on  OutDataTypeStr=Inherit: Same as first input
  Sum3 : Sum  Inputs=1  SaturateOnIntegerOverflow=on  InputSameDT=on  OutDataTypeStr=Inherit: Same as first input
  Terminator : Terminator
  Terminator1 : Terminator
  Urad*emissivity : Gain  Gain=5.6*emission_c  SaturateOnIntegerOverflow=on  OutDataTypeStr=Inherit: Same as input  ParamDataTypeStr=Inherit: Same as input
  active layers : Gain  Gain=active  SaturateOnIntegerOverflow=on  OutDataTypeStr=Inherit: Same as input  ParamDataTypeStr=Inherit: Same as input
  wallsurface : Gain  Gain=wallsurface  SaturateOnIntegerOverflow=on  OutDataTypeStr=Inherit: Same as input  ParamDataTypeStr=Inherit: Same as input
  qdots : Outport
  "[S]c" : Outport  Port=2
  wires:
  Math Function/1 -> Product1/3
  1-D Lookup Table/1 -> Product1/2  "coeff_upwards_downwards"
  Abs/1 -> Math Function/1
  Constant/1 -> Math Function/2
  active layers/1 -> Mux1/2
  Ground2/1 -> Mux1/3
  Mux1/1 -> "[S]c"/1
  Ground1/1 -> Mux1/5
  Ground/1 -> Mux1/1
  Sum3/1 -> active layers/1
  wallsurface/1 -> Sum3/1, Mux1/4  "[Qdotc, Qdotr]"
  Ts/1 -> Sum/2, Sum1/1  "Ts"
  Demux/2 -> Sum/1  "Tc"
  Mux/1 -> wallsurface/1
  Urad*emissivity/1 -> Mux/2, Sum2/2  "qdotr"
  Sum1/1 -> Urad*emissivity/1  "dTr"
  Demux/1 -> Terminator/1
  "[AIV]c"/1 -> Demux/1
  Demux/4 -> Terminator1/1
  Sum2/1 -> qdots/1
  Product1/1 -> Sum2/1, Mux/1  "qdotc"
  Sum/1 -> Product1/1, Abs/1, 1-D Lookup Table/1  "dTc"
  Demux/3 -> Sum1/2  "Tr"

== system carnot/Load/Houses/heat_transfer/alfa_floor ==
  note: dynamic, convective heat transfer coefficients according to: Glück B.: Wärmeübergangskoeffizienten an thermisch aktiven Bauteiloberflächen
      | und der Übergang zu Basiskennlinien für die Wärmestromdichte; gi Gesundheits-Ingenieur; 128. Jahrgang 2007, Heft 1, Seiten 1-10
  note: (°C)
  note: (W/m^2)
  note: Convective and radiative heat transfer at the SURFACE OF A HORIZONTAL FLOOR
  note: s: surface
      | c: convective
      | r: radiative
  note: CONVENTION:
      | Qdot > 0 and qdots < 0, if Ts > T (heat flows from wall surface to room node),
      | Qdot < 0 and qdots > 0, if Ts < T (heat flows from room node to wall surface).
  Ts : Inport
  "[AIV]f" : Inport  Port=2
  Qdot sol : Inport  Port=3
  1-D Lookup Table : Lookup_n-D  NumberOfTableDimensions=1  BreakpointsForDimension1=[-10 -0.01 0.01 10]  BeginIndexSearchUsingPreviousIndexResult=on  Table=[0.54 0.54 2 2]  InternalRulePriority=Speed  RndMeth=Simplest  InputSameDT=on
  1/wallsurface : Gain  Gain=1/wallsurface  SaturateOnIntegerOverflow=on  OutDataTypeStr=Inherit: Same as input  ParamDataTypeStr=Inherit: Same as input
  Abs : Abs
  Constant : Constant  Value=0.31
  Demux : Demux  Outputs=[1 1 1 6]
  Ground : Ground
  Ground1 : Ground
  Ground2 : Ground
  Math Function : Math  Operator=pow  SaturateOnIntegerOverflow=on
  Mux : Mux  Inputs=[1 1]
  Mux1 : Mux  Inputs=[4 1 1 2 5]
  Product1 : Product  Inputs=3  SaturateOnIntegerOverflow=on  RndMeth=Zero  InputSameDT=on  OutDataTypeStr=Inherit: Same as first input
  Sum : Sum  Inputs=-+  SaturateOnIntegerOverflow=on  InputSameDT=on  OutDataTypeStr=Inherit: Same as first input
  Sum1 : Sum  Inputs=+-  SaturateOnIntegerOverflow=on  InputSameDT=on  OutDataTypeStr=Inherit: Same as first input
  Sum2 : Sum  Inputs=+--  SaturateOnIntegerOverflow=on  InputSameDT=on  OutDataTypeStr=Inherit: Same as first input
  Sum3 : Sum  Inputs=1  SaturateOnIntegerOverflow=on  InputSameDT=on  OutDataTypeStr=Inherit: Same as first input
  Terminator : Terminator
  Terminator1 : Terminator
  Urad*emissivity : Gain  Gain=5.6*emission_f  SaturateOnIntegerOverflow=on  OutDataTypeStr=Inherit: Same as input  ParamDataTypeStr=Inherit: Same as input
  active? : Gain  Gain=active  SaturateOnIntegerOverflow=on  OutDataTypeStr=Inherit: Same as input  ParamDataTypeStr=Inherit: Same as input
  wallsurface : Gain  Gain=wallsurface  SaturateOnIntegerOverflow=on  OutDataTypeStr=Inherit: Same as input  ParamDataTypeStr=Inherit: Same as input
  qdots : Outport
  "[S]f" : Outport  Port=2
  wires:
  Sum/1 -> Product1/1, 1-D Lookup Table/1, Abs/1  "dTc"
  Constant/1 -> Math Function/2
  Abs/1 -> Math Function/1
  1-D Lookup Table/1 -> Product1/2  "coeff_upwards_downwards"
  Math Function/1 -> Product1/3
  Demux/3 -> Sum1/2  "Tr"
  Product1/1 -> Mux/1, Sum2/2  "qdotc"
  Mux/1 -> wallsurface/1
  Urad*emissivity/1 -> Sum2/3, Mux/2  "qdotr"
  Sum1/1 -> Urad*emissivity/1  "dTr"
  Demux/1 -> Terminator/1
  "[AIV]f"/1 -> Demux/1
  Demux/4 -> Terminator1/1
  1/wallsurface/1 -> Sum2/1
  Ts/1 -> Sum1/1, Sum/2  "Ts"
  Sum2/1 -> qdots/1
  Demux/2 -> Sum/1  "Tc"
  wallsurface/1 -> Mux1/4, Sum3/1  "[Qdotc, Qdotr]"
  Qdot sol/1 -> 1/wallsurface/1
  Sum3/1 -> active?/1
  Ground/1 -> Mux1/1
  Ground1/1 -> Mux1/5
  Mux1/1 -> "[S]f"/1
  Ground2/1 -> Mux1/3
  active?/1 -> Mux1/2

== system carnot/Load/Houses/heat_transfer/alfa_wall_in ==
  note: (°C)
  note: (W/m^2)
  note: Convective and radiative heat transfer at the INDOOR SURFACE of a VERTICAL OUTER WALL
  note: CONVENTION:
      | Qdot > 0 and qdots < 0, if Ts > T (heat flows from wall surface to room node),
      | Qdot < 0 and qdots > 0, if Ts < T (heat flows from room node to wall surface).
  note: s: surface
      | c: convective
      | r: radiative
  note: dynamic, convective heat transfer coefficients according to: Glück B.: Wärmeübergangskoeffizienten an thermisch aktiven Bauteiloberflächen
      | und der Übergang zu Basiskennlinien für die Wärmestromdichte; gi Gesundheits-Ingenieur; 128. Jahrgang 2007, Heft 1, Seiten 1-10
  Ts2 : Inport
  "[AIV]" : Inport  Port=2
  Abs : Abs
  Constant : Constant  Value=0.3
  Demux : Demux  Outputs=[1 1 1 6]
  Ground : Ground
  Ground1 : Ground
  Ground2 : Ground
  Math Function : Math  Operator=pow  SaturateOnIntegerOverflow=on
  Mux : Mux  Inputs=2
  Mux1 : Mux  Inputs=[4 1 1 2 5]
  Product1 : Product  SaturateOnIntegerOverflow=on  RndMeth=Zero  InputSameDT=on  OutDataTypeStr=Inherit: Same as first input
  Sum : Sum  Inputs=+-  SaturateOnIntegerOverflow=on  InputSameDT=on  OutDataTypeStr=Inherit: Same as first input
  Sum1 : Sum  Inputs=+-  SaturateOnIntegerOverflow=on  InputSameDT=on  OutDataTypeStr=Inherit: Same as first input
  Sum2 : Sum  Inputs=--  SaturateOnIntegerOverflow=on  InputSameDT=on  OutDataTypeStr=Inherit: Same as first input
  Sum3 : Sum  Inputs=1  SaturateOnIntegerOverflow=on  InputSameDT=on  OutDataTypeStr=Inherit: Same as first input
  Terminator : Terminator
  Terminator1 : Terminator
  Urad*emissivity : Gain  Gain=5.6*emission_in  SaturateOnIntegerOverflow=on  OutDataTypeStr=Inherit: Same as input  ParamDataTypeStr=Inherit: Same as input
  active layers : Gain  Gain=active  SaturateOnIntegerOverflow=on  OutDataTypeStr=Inherit: Same as input  ParamDataTypeStr=Inherit: Same as input
  gain : Gain  Gain=1.6  SaturateOnIntegerOverflow=on  OutDataTypeStr=Inherit: Same as input  ParamDataTypeStr=Inherit: Same as input
  wallsurface : Gain  Gain=wallsurface  SaturateOnIntegerOverflow=on  OutDataTypeStr=Inherit: Same as input  ParamDataTypeStr=Inherit: Same as input
  qdots2 : Outport
  "[S]" : Outport  Port=2
  wires:
  active layers/1 -> Mux1/2
  Ground2/1 -> Mux1/3
  Mux1/1 -> "[S]"/1
  Ground1/1 -> Mux1/5
  Ground/1 -> Mux1/1
  Sum3/1 -> active layers/1
  wallsurface/1 -> Sum3/1, Mux1/4  "[Qdotc, Qdotr]"
  Sum2/1 -> qdots2/1
  Demux/4 -> Terminator1/1
  "[AIV]"/1 -> Demux/1
  Demux/1 -> Terminator/1
  Demux/2 -> Sum/2  "Tc"
  Sum1/1 -> Urad*emissivity/1  "dTr"
  Urad*emissivity/1 -> Mux/2, Sum2/2  "qdotr"
  Mux/1 -> wallsurface/1
  Ts2/1 -> Sum/1, Sum1/1  "Ts"
  Demux/3 -> Sum1/2  "Tr"
  Product1/1 -> Sum2/1, Mux/1  "qdotc"
  Sum/1 -> Product1/1, Abs/1  "dTc"
  Constant/1 -> Math Function/2
  Abs/1 -> Math Function/1
  Math Function/1 -> gain/1
  gain/1 -> Product1/2

== system carnot/Load/Houses/heat_transfer/alfa_wall_out ==
  note: dynamic, convective heat transfer coefficients according to: Glück B.: Wärmeübergangskoeffizienten an thermisch aktiven Bauteiloberflächen
      | und der Übergang zu Basiskennlinien für die Wärmestromdichte; gi Gesundheits-Ingenieur; 128. Jahrgang 2007, Heft 1, Seiten 1-10
  note: Convective heat transfer outer surface according to EN 6946
      | Radiative heat transfer to the ground is limited by a view of 0.25, i.e. view factor to the sky is 0.75 (Frohner, 2005)
  note: Convective and radiative heat transfer at the WEATHER EXPOSED SURFACE OF AN OUTER WALL
  note: s: surface
      | c: convective
      | r: radiative
      | h: in height
      | t: tilted surface
  note: modified
      | weather data
  note: CONVENTION:
      | qdots < 0, if Ts > T, heat flows from window surface (resp. room node) to ambient,
      | qdots > 0, if Ts < T, heat flows from ambient to window surface (resp. room node).
  note: wind dependent heat transfer EN 6946
  WDB : Inport
  Ts1 : Inport  Port=2
  Bias : Bias  Bias=4
  Bus Selector : BusSelector  OutputSignals=Temperature_Ambient,Temperature_Sky_Radiation,Wind_Speed
  Gain : Gain  Gain=4
  Product2 : Product  SaturateOnIntegerOverflow=on  RndMeth=Zero  InputSameDT=on  OutDataTypeStr=Inherit: Same as first input
  Sum : Sum  Inputs=+-  SaturateOnIntegerOverflow=on  InputSameDT=on  OutDataTypeStr=Inherit: Same as first input
  Sum2 : Sum  Inputs=+++  SaturateOnIntegerOverflow=on  InputSameDT=on  OutDataTypeStr=Inherit: Same as first input
  absorption_out : Gain  Gain=absorption_out  SaturateOnIntegerOverflow=on  OutDataTypeStr=Inherit: Same as input  ParamDataTypeStr=Inherit: Same as input
  q rad : Subsystem
  wall_surfrad : carnot/Load/Houses/heat_transfer/wall_surfrad  pos=pos
  qdots1 : Outport
  wires:
  Gain/1 -> Bias/1
  Bus Selector/3 -> Gain/1  "<Wind_Speed>"
  Bus Selector/2 -> q rad/3(Tsky)  "<Temperature_Sky_Radiation>"
  Bus Selector/1 -> q rad/1(Tamb), Sum/1  "<Temperature_Ambient>"
  Sum/1 -> Product2/1  "dTc"
  WDB/1 -> wall_surfrad/1, Bus Selector/1
  Sum2/1 -> qdots1/1
  Ts1/1 -> Sum/2, q rad/2(Twall)  "Ts (outer wall surface)"
  wall_surfrad/1 -> absorption_out/1
  Bias/1 -> Product2/2  "alfa"
  absorption_out/1 -> Sum2/3  "qdot,sun"
  Product2/1 -> Sum2/1  "qdot_conv"
  q rad/1(qrad) -> Sum2/2  "qdot_rad"

== system carnot/Load/Houses/heat_transfer/alfa_window_in ==
  note: (W/m^2)
  note: CONVENTION:
      | Qdot > 0 and qdots < 0, if Ts > T (heat flows from wall surface to room node),
      | Qdot < 0 and qdots > 0, if Ts < T (heat flows from room node to wall surface).
  note: s: surface
      | c: convective
      | r: radiative
  note: WINDOW = FRAME + GLASS
  note: (W/m^2)
  note: Convective and radiative heat transfer at the INDOOR SURFACE OF A VERTICAL WINDOW
      | with 1-4 layers (each 3 ... 8 mm thick)
  note: (°C)
  Ts2 : Inport
  "[sun_t]" : Inport  Port=2
  "[AIV]" : Inport  Port=3
  " glass surface" : Gain  Gain=(1-frame)*wallsurface  SaturateOnIntegerOverflow=on  OutDataTypeStr=Inherit: Same as input  ParamDataTypeStr=Inherit: Same as input
  Demux : Demux  Outputs=[1 1 1 6]
  Demux1 : Demux  Outputs=[1 2]
  Ground : Ground
  Ground1 : Ground
  Irradiation into room : Subsystem
  Mux : Mux  Inputs=2
  Mux1 : Mux  Inputs=[1 5 2 5]
  Product6 : Product  SaturateOnIntegerOverflow=on  InputSameDT=on  OutDataTypeStr=Inherit: Same as first input
  Sum : Sum  Inputs=-+  SaturateOnIntegerOverflow=on  InputSameDT=on  OutDataTypeStr=Inherit: Same as first input
  Sum1 : Sum  Inputs=+-  SaturateOnIntegerOverflow=on  InputSameDT=on  OutDataTypeStr=Inherit: Same as first input
  Sum2 : Sum  Inputs=--  SaturateOnIntegerOverflow=on  InputSameDT=on  OutDataTypeStr=Inherit: Same as first input
  Sum3 : Sum  Inputs=1  SaturateOnIntegerOverflow=on  InputSameDT=on  OutDataTypeStr=Inherit: Same as first input
  Terminator : Terminator
  Terminator1 : Terminator
  Urad*emissivity : Gain  Gain=5.6*emission_in  SaturateOnIntegerOverflow=on  OutDataTypeStr=Inherit: Same as input  ParamDataTypeStr=Inherit: Same as input
  transmission coefficient 1-2-3-4-layer(s) : Subsystem
  u_convection : Gain  Gain=2.5  SaturateOnIntegerOverflow=on  OutDataTypeStr=Inherit: Same as input  ParamDataTypeStr=Inherit: Same as input
  u_rad1 : Constant  Value=zeros(numlayer,1)
  window surface : Gain  Gain=wallsurface  SaturateOnIntegerOverflow=on  OutDataTypeStr=Inherit: Same as input  ParamDataTypeStr=Inherit: Same as input
  qdots2 : Outport
  qdot_abs : Outport  Port=2
  "[S]" : Outport  Port=3
  wires:
  Sum3/1 -> Product6/1
  Product6/1 -> qdot_abs/1
  Ground1/1 -> Mux1/4
  Ground/1 -> Mux1/2
  Mux1/1 -> "[S]"/1
  Sum2/1 -> qdots2/1
  Demux/4 -> Terminator1/1
  "[AIV]"/1 -> Demux/1
  Demux/1 -> Terminator/1
  Mux/1 -> window surface/1
  Sum1/1 -> Urad*emissivity/1  "dTr"
  Ts2/1 -> Sum/2, Sum1/1  "Ts"
  Urad*emissivity/1 -> Sum2/2, Mux/2  "qdotr"
  u_convection/1 -> Mux/1, Sum2/1  "qdotc"
  Irradiation into room/1(qdot_sol) -> " glass surface"/1  "qdot_sol (>= 0)"
  Demux1/1 -> transmission coefficient 1-2-3-4-layer(s)/1(teta)  "teta"
  "[sun_t]"/1 -> Demux1/1
  " glass surface"/1 -> Mux1/1  "Qdot_sol"
  window surface/1 -> Mux1/3  "[Qdotc, Qdotr]"
  Demux/2 -> Sum/1  "Tc"
  u_rad1/1 -> Product6/2
  Sum/1 -> u_convection/1  "dTc"
  Demux/3 -> Sum1/2  "Tr"
  Demux1/2 -> Irradiation into room/2("[I_t]"), Sum3/1  "[I_t]"
  transmission coefficient 1-2-3-4-layer(s)/1("[tau]") -> Irradiation into room/1("[tau]")

== system carnot/Load/Houses/heat_transfer/alfa_window_out ==
  note: CONVENTION:
      | qdots < 0, if Ts > T, heat flows from window surface (resp. room node) to ambition,
      | qdots > 0, if Ts < T, heat flows from ambition to window surface (resp. room node).
  note: s: surface
      | c: convective
      | r: radiative
      | h: in height
      | t: tilted surface
  note: Convective and radiative heat transfer at the OUTDOOR SURFACE OF A VERTICAL WINDOW
  note: WINDOW = FRAME + GLASS
  WDB : Inport
  g : Inport  Port=2
  Ts1 : Inport  Port=3
  Bias : Bias  Bias=2.8
  Bus Selector : BusSelector  OutputSignals=Wind_Speed,Temperature_Ambient,Temperature_Sky_Radiation
  Bus Selector1 : BusSelector  OutputSignals=Incidence_Angle_sun,Solar_Radiation_direct_surface,Solar_Radiation_diffuse_surface
  Gain : Gain  Gain=3
  Mux1 : Mux  Inputs=2
  Mux2 : Mux  Inputs=2
  Product6 : Product  SaturateOnIntegerOverflow=on  InputSameDT=on  OutDataTypeStr=Inherit: Same as first input
  Product7 : Product  SaturateOnIntegerOverflow=on  InputSameDT=on  OutDataTypeStr=Inherit: Same as first input
  Radiation_on_Inclined_Surface : carnot/Weather/Radiation_on_Inclined_Surface  sky=Perez 1990  reflect=0.2
  Sum : Sum  Inputs=+-  SaturateOnIntegerOverflow=on  InputSameDT=on  OutDataTypeStr=Inherit: Same as first input
  Sum2 : Sum  Inputs=+++  SaturateOnIntegerOverflow=on  InputSameDT=on  OutDataTypeStr=Inherit: Same as first input
  Sum3 : Sum  SaturateOnIntegerOverflow=on  InputSameDT=on  OutDataTypeStr=Inherit: Same as first input
  absorption_out * frame : Gain  Gain=absorption_out * frame  SaturateOnIntegerOverflow=on  OutDataTypeStr=Inherit: Same as input  ParamDataTypeStr=Inherit: Same as input
  position : Constant  Value=pos
  wall_out_ IR_radiation : carnot/Load/Houses/heat_transfer/wall_out_ IR_radiation
  "[sun_t]" : Outport
  qdots1 : Outport  Port=2
  wires:
  Gain/1 -> Bias/1
  Bus Selector/1 -> Gain/1  "<Wind_Speed>"
  Bus Selector/3 -> wall_out_ IR_radiation/2  "<Temperature_Sky_Radiation>"
  Bus Selector/2 -> Sum/1, wall_out_ IR_radiation/1  "<Temperature_Ambient>"
  Bus Selector1/3 -> Sum3/2, Mux2/2  "<Solar_Radiation_diffuse_surface>"
  Mux2/1 -> Product6/1
  Product6/1 -> Mux1/2
  Sum/1 -> Product7/1  "dTc"
  WDB/1 -> Bus Selector/1, Radiation_on_Inclined_Surface/1
  Bus Selector1/1 -> Mux1/1  "<Incidence_Angle_sun>"
  Sum3/1 -> absorption_out * frame/1
  Sum2/1 -> qdots1/1
  g/1 -> Product6/2
  absorption_out * frame/1 -> Sum2/3
  Bus Selector1/2 -> Sum3/1, Mux2/1  "<Solar_Radiation_direct_surface>"
  Mux1/1 -> "[sun_t]"/1
  Ts1/1 -> wall_out_ IR_radiation/3, Sum/2  "Ts (outer wall surface)"
  wall_out_ IR_radiation/1 -> Sum2/2  "qdotr"
  Bias/1 -> Product7/2  "alfa"
  Product7/1 -> Sum2/1  "qdot,conv"
  position/1 -> Radiation_on_Inclined_Surface/2
  Radiation_on_Inclined_Surface/1 -> Bus Selector1/1

== system carnot/Load/Houses/heat_transfer/wall_out_IR_radiation ==
  note: Wall has a view on 50% ground and 50% sky (true for vertical walls).
      | Longwave radiation emissiviy of ground and sky assumed to be 1.
  Tamb : Inport
  Tsky : Inport  Port=2
  Twall : Inport  Port=3
  Bias : Bias  Bias=273.15
  Gain : Gain  Gain=[-1 0.5 0.5]*emission_out*5.67e-8
  Math Function : Math  Operator=square  SaturateOnIntegerOverflow=on
  Math Function1 : Math  Operator=square  SaturateOnIntegerOverflow=on
  Mux : Mux  Inputs=3
  Sum : Sum  Inputs=1  SaturateOnIntegerOverflow=on  InputSameDT=on  OutDataTypeStr=Inherit: Same as first input
  qrad : Outport
  wires:
  Tsky/1 -> Mux/2
  Tamb/1 -> Mux/3
  Sum/1 -> qrad/1
  Twall/1 -> Mux/1
  Bias/1 -> Math Function/1
  Mux/1 -> Bias/1
  Math Function/1 -> Math Function1/1
  Gain/1 -> Sum/1
  Math Function1/1 -> Gain/1
